simulink model "sim_RCL"  (R2024b)
settings: Solver=VariableStepAuto  StartTime=0.0  StopTime=0.02  MaxStep=10e-6  RelTol=1e-3
settings Model: Creator=Sveta  LastModifiedBy=SvetlanaMeissner
settings SolverCC: AlgebraicLoopSolver=TrustRegion
settings DataIOCC: ReturnWorkspaceOutputs=off
settings DebuggingCC: UnconnectedInputMsg=warning  UnconnectedOutputMsg=warning  UnconnectedLineMsg=warning  ArithmeticOperatorsInVariantConditions=warning
settings ModelReferenceCC: EnableRefExpFcnMdlSchedulingChecks=on
settings SFSimCC: SimUseLocalCustomCode=off  CustomCodeUndefinedFunction=UseInterfaceOnly
settings RTWCC: RTWUseLocalCustomCode=off  GPUComputeCapability=3.5  DLArmComputeVersion=19.05
settings CodeAppCC: StateflowObjectComments=on

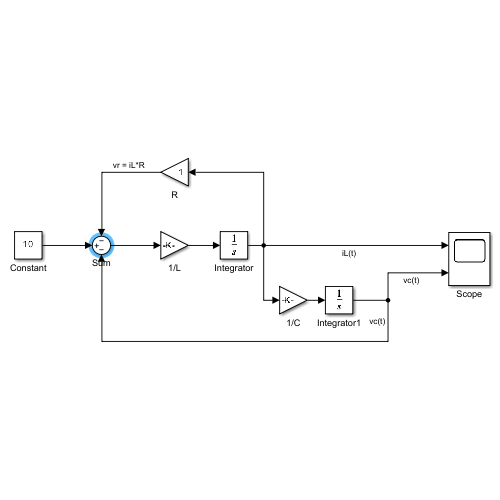
[thumbnail: Simulink's stored preview of the top-level diagram]
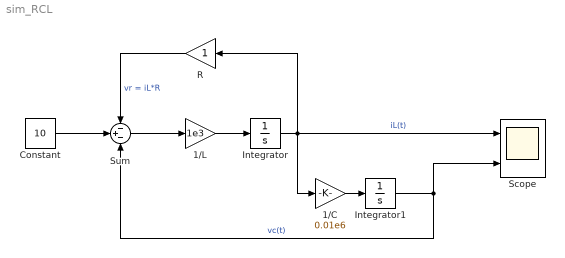
== system sim_RCL ==
  1/C : Gain  Gain=0.01e6
  1/L : Gain  Gain=1e3
  Constant : Constant  Value=10
  Integrator : Integrator
  Integrator1 : Integrator
  R : Gain
  Scope : Scope  NumInputPorts=2
  Sum : Sum  Inputs=-+-
  wires:
  Constant/1 -> Sum/2
  Sum/1 -> 1/L/1
  1/L/1 -> Integrator/1
  Integrator/1 -> R/1, Scope/1, 1/C/1  "iL(t)"
  1/C/1 -> Integrator1/1
  Integrator1/1 -> Sum/3, Scope/2  "vc(t)"
  R/1 -> Sum/1  "vr = iL*R"
